simulink model "model_upr"  (R2024a)
settings: Solver=VariableStepAuto  StartTime=0.0  StopTime=10.0  RelTol=1e-3
settings Model: Creator=eva  LastModifiedBy=eva

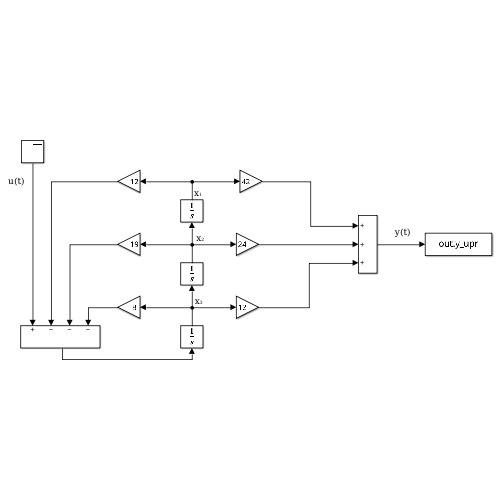
[thumbnail: Simulink's stored preview of the top-level diagram]
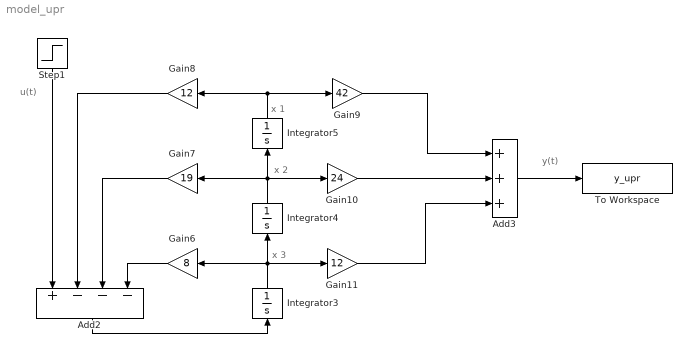
== system model_upr ==
  note: x 1
  note: x 2
  note: x 3
  note: u(t)
  note: y(t)
  Add2 : Sum  Inputs=+---
  Add3 : Sum  Inputs=+++
  Gain10 : Gain  Gain=24
  Gain11 : Gain  Gain=12
  Gain6 : Gain  Gain=8
  Gain7 : Gain  Gain=19
  Gain8 : Gain  Gain=12
  Gain9 : Gain  Gain=42
  Integrator3 : Integrator
  Integrator4 : Integrator
  Integrator5 : Integrator
  Step1 : Step  Time=0  SampleTime=0
  To Workspace : ToWorkspace  VariableName=y_upr  SaveFormat=Structure With Time  SampleTime=-1
  wires:
  Integrator3/1 -> Gain6/1, Integrator4/1, Gain11/1
  Integrator5/1 -> Gain9/1, Gain8/1
  Gain11/1 -> Add3/3
  Gain10/1 -> Add3/2
  Gain9/1 -> Add3/1
  Integrator4/1 -> Gain7/1, Gain10/1, Integrator5/1
  Gain6/1 -> Add2/4
  Gain7/1 -> Add2/3
  Gain8/1 -> Add2/2
  Step1/1 -> Add2/1
  Add3/1 -> To Workspace/1
  Add2/1 -> Integrator3/1
